simulink model "SistemaCompleto_PMSM"  (R2023b)
settings: Solver=VariableStepAuto  StartTime=0.0  StopTime=2  RelTol=1e-3
PostLoadFcn:
  | parametros_sistema_completo
  | run("parametros_sistema_completo.mlx")
values from neighbouring files (symbols this model uses):
  a_cu = 3.9e-3    (= 0.0039)    [parametros_sistema_completo.m]    (also in workspace_params.mat)
  A_i = [0,  1,                          0 ... (first row only)    [analisis_estabilidad_LA.m]
  b_eq = params.b_total    [calcular_matriz_AO.m]    (also in calculo_incertidumbre_y_control.m = b_m + b_l/(r^2); parametros_sistema_completo.m = 2.19444444444e-05; workspace_params.mat = 2.19444444444e-05)
  C_ts = C_ts * (1 + tol_pct)    [calculo_incertidumbre_y_control.m]    (also in parametros_sistema_completo.m = 0.818; workspace_params.mat = 0.818)
  g = 9.80665    [parametros_sistema_completo.m]    (also in workspace_params.mat)
  J_eq = params.J_total    [calcular_matriz_AO.m]    (also in calculo_incertidumbre_y_control.m = J_m + J_l/r^2; parametros_sistema_completo.m = 1.97847222222e-05; workspace_params.mat = 3.28055555556e-05)
  k_l = m*l_cm + m_l*l_l    [calculo_incertidumbre_y_control.m]    (also in parametros_sistema_completo.m = 0.25; workspace_params.mat = 0.625)
  L_d = L_d    * (1 - tol_pct)    [calculo_incertidumbre_y_control.m]    (also in parametros_sistema_completo.m = 0.0066; workspace_params.mat = 0.0066)
  L_ls = L_ls   * (1 - tol_pct)    [calculo_incertidumbre_y_control.m]    (also in parametros_sistema_completo.m = 0.0008; workspace_params.mat = 0.0008)
  L_q = L_q    * (1 - tol_pct)    [calculo_incertidumbre_y_control.m]    (also in parametros_sistema_completo.m = 0.0058; workspace_params.mat = 0.0058)
  lambda_r = lambda_r * (1 + tol_pct)    [calculo_incertidumbre_y_control.m]    (also in parametros_sistema_completo.m = 0.016; workspace_params.mat = 0.016)
  P_p = 3    [parametros_sistema_completo.m]    (also in workspace_params.mat)
  params = struct()    [evaluar_migracion_Ids.m]    (also in parametros_sistema_completo.m; workspace_params.mat = )
  r = params.r_red    [calcular_matriz_AO.m]    (also in parametros_sistema_completo.m = 120; workspace_params.mat = 120)
  R_s_sim = R_sREF * (1 + a_cu * (T_s_sim - T_sREF))    [configurar_temperatura_516.m]
  R_sREF = R_sREF * (1 - tol_pct)    [calculo_incertidumbre_y_control.m]    (also in parametros_sistema_completo.m = 1.02; workspace_params.mat = 1.02)
  R_ts_amb = R_ts_amb * (1 - tol_pct)    [calculo_incertidumbre_y_control.m]    (also in parametros_sistema_completo.m = 146.7; workspace_params.mat = 146.7)
  T_amb = 20    [parametros_sistema_completo.m]    (also in workspace_params.mat)
  T_s = x(6)    [modulador_torque_521.m]    (also in simulacion_dinamica_516.m)
  T_sREF = 20    [parametros_sistema_completo.m]    (also in workspace_params.mat)
undefined symbols (not defined in the file or in its folder): A_T, A_theta, A_v, b_a, B_i, B_T, B_theta, B_v, C_i, C_T, C_theta, C_v, consigna_posicion, D_i, D_T, D_theta, D_v, i_ds_inicial, Is_pico, Is_rms_max, Is_rms_nom, K_e_i_m_int, K_e_tita_m, K_e_tita_m_int, K_e_w_m, K_e_w_m_int, K_p0, K_pd, K_pq, K_sa, K_sia, pos_inicial, t_rampa_acel, t_rampa_vel, V_sl_max, x0_ias, x0_ibs, x0_ics, x0_T, x0_theta
libraries: simulink_extras x8, SignalEditorBlockLib x6, eeStairGenerator x4, simulink x1
(part 5 of 7)

== system SistemaCompleto_PMSM/Modelo Global NL Controlador modulador de torque3/Planta/Subsistema Electromagnetico ==
  v_qs : Inport
  v_ds : Inport  Port=2
  v_0s : Inport  Port=3
  ωm : Inport  Port=4
  R_s(T(t)) : Inport  Port=5
  Add : Sum  Inputs=-++
  Add1 : Sum  Inputs=--+
  Add2 : Sum  Inputs=|-+
  Add3 : Sum  Inputs=|++
  Gain : Gain  Gain=1/L_q
  Gain1 : Gain  Gain=1/L_d
  Gain2 : Gain  Gain=1/L_ls
  Gain3 : Gain  Gain=P_p
  Gain4 : Gain  Gain=L_d
  Gain5 : Gain  Gain=L_q
  Gain6 : Gain  Gain=3/2*P_p
  Gain7 : Gain  Gain=L_d-L_q
  Integrator : Integrator
  Integrator1 : Integrator  InitialCondition=i_ds_inicial
  Integrator2 : Integrator
  Product{,1..6} (7 alike) : Product
  Sum3 : Sum  Inputs=|++
  λ : Constant  Value=lambda_r
  i_qs : Outport
  i_ds : Outport  Port=2
  i_0s : Outport  Port=3
  T_m : Outport  Port=4
  wires:
  v_0s/1 -> Add2/2
  Gain5/1 -> Add/3
  Gain3/1 -> Product4/2, Product3/1  "ωr"
  Integrator/1 -> Product4/1, Product/2, i_qs/1, Product5/1, Product6/1
  v_qs/1 -> Add1/3
  R_s(T(t))/1 -> Product2/2, Product1/1, Product/1
  Gain4/1 -> Sum3/1
  Product1/1 -> Add/1
  Integrator2/1 -> i_0s/1, Product2/1
  Sum3/1 -> Product3/2
  Integrator1/1 -> Gain4/1, Product1/2, i_ds/1, Product6/2
  Product/1 -> Add1/2
  Product4/1 -> Gain5/1
  ωm/1 -> Gain3/1
  Add3/1 -> Gain6/1
  Gain/1 -> Integrator/1
  Gain6/1 -> T_m/1
  Product2/1 -> Add2/1
  λ/1 -> Sum3/2, Product5/2
  Gain1/1 -> Integrator1/1
  Add/1 -> Gain1/1
  Add1/1 -> Gain/1
  Product6/1 -> Gain7/1
  Product3/1 -> Add1/1
  Gain2/1 -> Integrator2/1
  Gain7/1 -> Add3/2
  v_ds/1 -> Add/2
  Add2/1 -> Gain2/1
  Product5/1 -> Add3/1

== system SistemaCompleto_PMSM/Modelo Global NL Controlador modulador de torque3/Planta/Subsistema Mecanico ==
  Tld(t)[N.m] : Inport
  Tm(t)[N.m] : Inport  Port=2
  1/J_eq[kg.m2] : Gain  Gain=1/J_eq
  Gain : Gain  Gain=1/r
  Gain1 : Gain  Gain=1/r
  Integrator : Integrator  InitialCondition=pos_inicial*r
  Integrator1 : Integrator
  Sin : Trigonometry
  Sum : Sum  Inputs=-+-
  Sum1 : Sum
  "[N.m/rad]" : Gain  Gain=g*k_l
  b_eq[N.m/rad/s] : Gain  Gain=b_eq
  θm(t) : Outport
  ωm(t) : Outport  Port=2
  wires:
  Gain1/1 -> Sin/1
  Sin/1 -> "[N.m/rad]"/1  "θm[rad]"
  Integrator1/1 -> Integrator/1, ωm(t)/1, b_eq[N.m/rad/s]/1  "ωm[rad/s]"
  Tld(t)[N.m]/1 -> Sum1/1
  b_eq[N.m/rad/s]/1 -> Sum/3
  1/J_eq[kg.m2]/1 -> Integrator1/1  "dω/dt [rad/s^2]"
  Gain/1 -> Sum/1
  "[N.m/rad]"/1 -> Sum1/2
  Integrator/1 -> θm(t)/1, Gain1/1  "θm[rad]"
  Sum/1 -> 1/J_eq[kg.m2]/1
  Tm(t)[N.m]/1 -> Sum/2
  Sum1/1 -> Gain/1

== system SistemaCompleto_PMSM/Modelo Global NL Controlador modulador de torque3/Planta/Subsistema Térmico ==
  i_qs2 : Inport
  i_ds2 : Inport  Port=2
  i_0s2 : Inport  Port=3
  Add : Sum  Inputs=+-
  Add1 : Sum
  Add2 : Sum  Inputs=+++
  Add3 : Sum  Inputs=+-
  Add4 : Sum  Inputs=-+
  Constant : Constant  Value=T_sREF
  Constant1 : Constant
  Constant2 : Constant  Value=T_amb
  Gain : Gain  Gain=R_sREF
  Gain1 : Gain  Gain=a_cu
  Gain2 : Gain  Gain=3/2
  Gain3 : Gain  Gain=2
  Gain4 : Gain  Gain=1/C_ts
  Gain5 : Gain  Gain=1/R_ts_amb
  Integrator : Integrator  InitialCondition=20
  Product : Product
  Square : Math  Operator=square  OutDataTypeStr=double
  Square1 : Math  Operator=square
  Square2 : Math  Operator=square
  R_s : Outport
  T_s : Outport  Port=2
  wires:
  Constant1/1 -> Add1/2
  Constant/1 -> Add/2
  i_qs2/1 -> Square/1
  Gain/1 -> R_s/1, Product/1
  Square/1 -> Add2/1
  Add2/1 -> Gain2/1
  Constant2/1 -> Add4/1
  i_ds2/1 -> Square1/1
  Gain5/1 -> Add3/2
  Integrator/1 -> Add4/2, T_s/1, Add/1  "T_s"
  Add1/1 -> Gain/1
  i_0s2/1 -> Square2/1
  Square1/1 -> Add2/2
  Product/1 -> Add3/1  "Ps_Perd"
  Gain2/1 -> Product/2
  Add/1 -> Gain1/1
  Square2/1 -> Gain3/1
  Gain1/1 -> Add1/1
  Add3/1 -> Gain4/1
  Add4/1 -> Gain5/1
  Gain3/1 -> Add2/3
  Gain4/1 -> Integrator/1

== system SistemaCompleto_PMSM/Modelo Global NL Controlador modulador de torque3/Planta/TI de Park ==
  f_q : Inport
  f_d : Inport  Port=2
  f_0 : Inport  Port=3
  θ_r : Inport  Port=4
  Add : Sum  Inputs=+++
  Add1 : Sum  Inputs=+-
  Add2 : Sum
  Add3 : Sum  Inputs=+++
  Add4 : Sum  Inputs=+++
  Constant : Constant  Value=2/3*pi
  Constant1 : Constant  Value=2/3*pi
  Cos : Trigonometry  Operator=cos
  Cos1 : Trigonometry
  Cos2 : Trigonometry  Operator=cos
  Cos3 : Trigonometry  Operator=cos
  Cos4 : Trigonometry
  Cos5 : Trigonometry
  Product{,1..5} (6 alike) : Product
  f_a : Outport
  f_b : Outport  Port=2
  f_c : Outport  Port=3
  wires:
  Product4/1 -> Add3/2
  Cos1/1 -> Product1/1
  Cos/1 -> Product/1
  Product1/1 -> Add/2
  Add3/1 -> f_b/1
  Cos3/1 -> Product3/1
  Product3/1 -> Add3/1
  f_d/1 -> Product1/2, Product5/2, Product4/2
  Constant1/1 -> Add2/2
  Constant/1 -> Add1/2
  f_0/1 -> Add3/3, Add4/3, Add/3
  Add1/1 -> Cos3/1, Cos4/1
  Product/1 -> Add/1
  f_q/1 -> Product/2, Product2/2, Product3/2
  Cos4/1 -> Product4/1
  θ_r/1 -> Add2/1, Add1/1, Cos/1, Cos1/1
  Add/1 -> f_a/1
  Add4/1 -> f_c/1
  Cos2/1 -> Product2/1
  Cos5/1 -> Product5/1
  Add2/1 -> Cos5/1, Cos2/1
  Product2/1 -> Add4/1
  Product5/1 -> Add4/2

== system SistemaCompleto_PMSM/Modelo Global NL Controlador modulador de torque3/Planta/Transformacion de Park ==
  f_a : Inport
  f_b : Inport  Port=2
  f_c : Inport  Port=3
  θ_r : Inport  Port=4
  Add : Sum  Inputs=+++
  Add1 : Sum  Inputs=+-
  Add2 : Sum
  Add3 : Sum  Inputs=+++
  Add4 : Sum  Inputs=+++
  Constant : Constant  Value=2/3*pi
  Constant1 : Constant  Value=2/3*pi
  Cos : Trigonometry  Operator=cos
  Cos1 : Trigonometry  Operator=cos
  Cos2 : Trigonometry  Operator=cos
  Cos3 : Trigonometry
  Cos4 : Trigonometry
  Cos5 : Trigonometry
  Gain1 : Gain  Gain=2/3
  Gain2 : Gain  Gain=2/3
  Gain3 : Gain  Gain=1/3
  Product{,1..5} (6 alike) : Product
  f_q : Outport
  f_d : Outport  Port=2
  f_0 : Outport  Port=3
  wires:
  Cos5/1 -> Product5/1
  Gain2/1 -> f_q/1
  Product5/1 -> Add3/3
  Add/1 -> Gain2/1
  θ_r/1 -> Cos3/1, Cos/1, Add1/1, Add2/1
  Cos4/1 -> Product4/1
  Cos2/1 -> Product2/1
  f_a/1 -> Add4/3, Product3/2, Product/2
  Product/1 -> Add/1
  Add1/1 -> Cos1/1, Cos4/1
  f_c/1 -> Product2/2, Product5/2, Add4/1
  Constant/1 -> Add1/2
  Constant1/1 -> Add2/2
  f_b/1 -> Product1/2, Product4/2, Add4/2
  Add2/1 -> Cos2/1, Cos5/1
  Add4/1 -> Gain3/1
  Product3/1 -> Add3/1
  Product2/1 -> Add/3
  Gain3/1 -> f_0/1
  Cos3/1 -> Product3/1
  Add3/1 -> Gain1/1
  Gain1/1 -> f_d/1
  Product1/1 -> Add/2
  Cos/1 -> Product/1
  Cos1/1 -> Product1/1
  Product4/1 -> Add3/2

== system SistemaCompleto_PMSM/Modelo Global NL Controlador modulador de torque4/Planta/Subsistema Electromagnetico ==
  v_qs : Inport
  v_ds : Inport  Port=2
  v_0s : Inport  Port=3
  ωm : Inport  Port=4
  R_s(T(t)) : Inport  Port=5
  Add : Sum  Inputs=-++
  Add1 : Sum  Inputs=--+
  Add2 : Sum  Inputs=|-+
  Add3 : Sum  Inputs=|++
  Gain : Gain  Gain=1/L_q
  Gain1 : Gain  Gain=1/L_d
  Gain2 : Gain  Gain=1/L_ls
  Gain3 : Gain  Gain=P_p
  Gain4 : Gain  Gain=L_d
  Gain5 : Gain  Gain=L_q
  Gain6 : Gain  Gain=3/2*P_p
  Gain7 : Gain  Gain=L_d-L_q
  Integrator : Integrator
  Integrator1 : Integrator  InitialCondition=i_ds_inicial
  Integrator2 : Integrator
  Product{,1..6} (7 alike) : Product
  Sum3 : Sum  Inputs=|++
  λ : Constant  Value=lambda_r
  i_qs : Outport
  i_ds : Outport  Port=2
  i_0s : Outport  Port=3
  T_m : Outport  Port=4
  wires:
  v_0s/1 -> Add2/2
  Gain5/1 -> Add/3
  Gain3/1 -> Product4/2, Product3/1  "ωr"
  Integrator/1 -> Product4/1, Product/2, i_qs/1, Product5/1, Product6/1
  v_qs/1 -> Add1/3
  R_s(T(t))/1 -> Product2/2, Product1/1, Product/1
  Gain4/1 -> Sum3/1
  Product1/1 -> Add/1
  Integrator2/1 -> i_0s/1, Product2/1
  Sum3/1 -> Product3/2
  Integrator1/1 -> Gain4/1, Product1/2, i_ds/1, Product6/2
  Product/1 -> Add1/2
  Product4/1 -> Gain5/1
  ωm/1 -> Gain3/1
  Add3/1 -> Gain6/1
  Gain/1 -> Integrator/1
  Gain6/1 -> T_m/1
  Product2/1 -> Add2/1
  λ/1 -> Sum3/2, Product5/2
  Gain1/1 -> Integrator1/1
  Add/1 -> Gain1/1
  Add1/1 -> Gain/1
  Product6/1 -> Gain7/1
  Product3/1 -> Add1/1
  Gain2/1 -> Integrator2/1
  Gain7/1 -> Add3/2
  v_ds/1 -> Add/2
  Add2/1 -> Gain2/1
  Product5/1 -> Add3/1

== system SistemaCompleto_PMSM/Modelo Global NL Controlador modulador de torque4/Planta/Subsistema Mecanico ==
  Tld(t)[N.m] : Inport
  Tm(t)[N.m] : Inport  Port=2
  1/J_eq[kg.m2] : Gain  Gain=1/J_eq
  Gain : Gain  Gain=1/r
  Gain1 : Gain  Gain=1/r
  Integrator : Integrator  InitialCondition=pos_inicial*r
  Integrator1 : Integrator
  Sin : Trigonometry
  Sum : Sum  Inputs=-+-
  Sum1 : Sum
  "[N.m/rad]" : Gain  Gain=g*k_l
  b_eq[N.m/rad/s] : Gain  Gain=b_eq
  θm(t) : Outport
  ωm(t) : Outport  Port=2
  wires:
  Gain1/1 -> Sin/1
  Sin/1 -> "[N.m/rad]"/1  "θm[rad]"
  Integrator1/1 -> Integrator/1, ωm(t)/1, b_eq[N.m/rad/s]/1  "ωm[rad/s]"
  Tld(t)[N.m]/1 -> Sum1/1
  b_eq[N.m/rad/s]/1 -> Sum/3
  1/J_eq[kg.m2]/1 -> Integrator1/1  "dω/dt [rad/s^2]"
  Gain/1 -> Sum/1
  "[N.m/rad]"/1 -> Sum1/2
  Integrator/1 -> θm(t)/1, Gain1/1  "θm[rad]"
  Sum/1 -> 1/J_eq[kg.m2]/1
  Tm(t)[N.m]/1 -> Sum/2
  Sum1/1 -> Gain/1

== system SistemaCompleto_PMSM/Modelo Global NL Controlador modulador de torque4/Planta/Subsistema Térmico ==
  i_qs2 : Inport
  i_ds2 : Inport  Port=2
  i_0s2 : Inport  Port=3
  Add : Sum  Inputs=+-
  Add1 : Sum
  Add2 : Sum  Inputs=+++
  Add3 : Sum  Inputs=+-
  Add4 : Sum  Inputs=-+
  Constant : Constant  Value=T_sREF
  Constant1 : Constant
  Constant2 : Constant  Value=T_amb
  Gain : Gain  Gain=R_sREF
  Gain1 : Gain  Gain=a_cu
  Gain2 : Gain  Gain=3/2
  Gain3 : Gain  Gain=2
  Gain4 : Gain  Gain=1/C_ts
  Gain5 : Gain  Gain=1/R_ts_amb
  Integrator : Integrator  InitialCondition=20
  Product : Product
  Square : Math  Operator=square  OutDataTypeStr=double
  Square1 : Math  Operator=square
  Square2 : Math  Operator=square
  R_s : Outport
  T_s : Outport  Port=2
  wires:
  Constant1/1 -> Add1/2
  Constant/1 -> Add/2
  i_qs2/1 -> Square/1
  Gain/1 -> R_s/1, Product/1
  Square/1 -> Add2/1
  Add2/1 -> Gain2/1
  Constant2/1 -> Add4/1
  i_ds2/1 -> Square1/1
  Gain5/1 -> Add3/2
  Integrator/1 -> Add4/2, T_s/1, Add/1  "T_s"
  Add1/1 -> Gain/1
  i_0s2/1 -> Square2/1
  Square1/1 -> Add2/2
  Product/1 -> Add3/1  "Ps_Perd"
  Gain2/1 -> Product/2
  Add/1 -> Gain1/1
  Square2/1 -> Gain3/1
  Gain1/1 -> Add1/1
  Add3/1 -> Gain4/1
  Add4/1 -> Gain5/1
  Gain3/1 -> Add2/3
  Gain4/1 -> Integrator/1

== system SistemaCompleto_PMSM/Modelo Global NL Controlador modulador de torque4/Planta/TI de Park ==
  f_q : Inport
  f_d : Inport  Port=2
  f_0 : Inport  Port=3
  θ_r : Inport  Port=4
  Add : Sum  Inputs=+++
  Add1 : Sum  Inputs=+-
  Add2 : Sum
  Add3 : Sum  Inputs=+++
  Add4 : Sum  Inputs=+++
  Constant : Constant  Value=2/3*pi
  Constant1 : Constant  Value=2/3*pi
  Cos : Trigonometry  Operator=cos
  Cos1 : Trigonometry
  Cos2 : Trigonometry  Operator=cos
  Cos3 : Trigonometry  Operator=cos
  Cos4 : Trigonometry
  Cos5 : Trigonometry
  Product{,1..5} (6 alike) : Product
  f_a : Outport
  f_b : Outport  Port=2
  f_c : Outport  Port=3
  wires:
  Product4/1 -> Add3/2
  Cos1/1 -> Product1/1
  Cos/1 -> Product/1
  Product1/1 -> Add/2
  Add3/1 -> f_b/1
  Cos3/1 -> Product3/1
  Product3/1 -> Add3/1
  f_d/1 -> Product1/2, Product5/2, Product4/2
  Constant1/1 -> Add2/2
  Constant/1 -> Add1/2
  f_0/1 -> Add3/3, Add4/3, Add/3
  Add1/1 -> Cos3/1, Cos4/1
  Product/1 -> Add/1
  f_q/1 -> Product/2, Product2/2, Product3/2
  Cos4/1 -> Product4/1
  θ_r/1 -> Add2/1, Add1/1, Cos/1, Cos1/1
  Add/1 -> f_a/1
  Add4/1 -> f_c/1
  Cos2/1 -> Product2/1
  Cos5/1 -> Product5/1
  Add2/1 -> Cos5/1, Cos2/1
  Product2/1 -> Add4/1
  Product5/1 -> Add4/2

== system SistemaCompleto_PMSM/Modelo Global NL Controlador modulador de torque4/Planta/Transformacion de Park ==
  f_a : Inport
  f_b : Inport  Port=2
  f_c : Inport  Port=3
  θ_r : Inport  Port=4
  Add : Sum  Inputs=+++
  Add1 : Sum  Inputs=+-
  Add2 : Sum
  Add3 : Sum  Inputs=+++
  Add4 : Sum  Inputs=+++
  Constant : Constant  Value=2/3*pi
  Constant1 : Constant  Value=2/3*pi
  Cos : Trigonometry  Operator=cos
  Cos1 : Trigonometry  Operator=cos
  Cos2 : Trigonometry  Operator=cos
  Cos3 : Trigonometry
  Cos4 : Trigonometry
  Cos5 : Trigonometry
  Gain1 : Gain  Gain=2/3
  Gain2 : Gain  Gain=2/3
  Gain3 : Gain  Gain=1/3
  Product{,1..5} (6 alike) : Product
  f_q : Outport
  f_d : Outport  Port=2
  f_0 : Outport  Port=3
  wires:
  Cos5/1 -> Product5/1
  Gain2/1 -> f_q/1
  Product5/1 -> Add3/3
  Add/1 -> Gain2/1
  θ_r/1 -> Cos3/1, Cos/1, Add1/1, Add2/1
  Cos4/1 -> Product4/1
  Cos2/1 -> Product2/1
  f_a/1 -> Add4/3, Product3/2, Product/2
  Product/1 -> Add/1
  Add1/1 -> Cos1/1, Cos4/1
  f_c/1 -> Product2/2, Product5/2, Add4/1
  Constant/1 -> Add1/2
  Constant1/1 -> Add2/2
  f_b/1 -> Product1/2, Product4/2, Add4/2
  Add2/1 -> Cos2/1, Cos5/1
  Add4/1 -> Gain3/1
  Product3/1 -> Add3/1
  Product2/1 -> Add/3
  Gain3/1 -> f_0/1
  Cos3/1 -> Product3/1
  Add3/1 -> Gain1/1
  Gain1/1 -> f_d/1
  Product1/1 -> Add/2
  Cos/1 -> Product/1
  Cos1/1 -> Product1/1
  Product4/1 -> Add3/2

== system SistemaCompleto_PMSM/Modelo Global NL perfil trapezoidal aceleracion/Planta/Subsistema Electromagnetico ==
  v_qs : Inport
  v_ds : Inport  Port=2
  v_0s : Inport  Port=3
  ωm : Inport  Port=4
  R_s(T(t)) : Inport  Port=5
  Add : Sum  Inputs=-++
  Add1 : Sum  Inputs=--+
  Add2 : Sum  Inputs=|-+
  Add3 : Sum  Inputs=|++
  Gain : Gain  Gain=1/L_q
  Gain1 : Gain  Gain=1/L_d
  Gain2 : Gain  Gain=1/L_ls
  Gain3 : Gain  Gain=P_p
  Gain4 : Gain  Gain=L_d
  Gain5 : Gain  Gain=L_q
  Gain6 : Gain  Gain=3/2*P_p
  Gain7 : Gain  Gain=L_d-L_q
  Integrator : Integrator
  Integrator1 : Integrator  InitialCondition=i_ds_inicial
  Integrator2 : Integrator
  Product{,1..6} (7 alike) : Product
  Sum3 : Sum  Inputs=|++
  λ : Constant  Value=lambda_r
  i_qs : Outport
  i_ds : Outport  Port=2
  i_0s : Outport  Port=3
  T_m : Outport  Port=4
  wires:
  v_0s/1 -> Add2/2
  Gain5/1 -> Add/3
  Gain3/1 -> Product4/2, Product3/1  "ωr"
  Integrator/1 -> Product4/1, Product/2, i_qs/1, Product5/1, Product6/1
  v_qs/1 -> Add1/3
  R_s(T(t))/1 -> Product2/2, Product1/1, Product/1
  Gain4/1 -> Sum3/1
  Product1/1 -> Add/1
  Integrator2/1 -> i_0s/1, Product2/1
  Sum3/1 -> Product3/2
  Integrator1/1 -> Gain4/1, Product1/2, i_ds/1, Product6/2
  Product/1 -> Add1/2
  Product4/1 -> Gain5/1
  ωm/1 -> Gain3/1
  Add3/1 -> Gain6/1
  Gain/1 -> Integrator/1
  Gain6/1 -> T_m/1
  Product2/1 -> Add2/1
  λ/1 -> Sum3/2, Product5/2
  Gain1/1 -> Integrator1/1
  Add/1 -> Gain1/1
  Add1/1 -> Gain/1
  Product6/1 -> Gain7/1
  Product3/1 -> Add1/1
  Gain2/1 -> Integrator2/1
  Gain7/1 -> Add3/2
  v_ds/1 -> Add/2
  Add2/1 -> Gain2/1
  Product5/1 -> Add3/1

== system SistemaCompleto_PMSM/Modelo Global NL perfil trapezoidal aceleracion/Planta/Subsistema Mecanico ==
  Tld(t)[N.m] : Inport
  Tm(t)[N.m] : Inport  Port=2
  1/J_eq[kg.m2] : Gain  Gain=1/J_eq
  Gain : Gain  Gain=1/r
  Gain1 : Gain  Gain=1/r
  Integrator : Integrator  InitialCondition=pos_inicial*r
  Integrator1 : Integrator
  Sin : Trigonometry
  Sum : Sum  Inputs=-+-
  Sum1 : Sum
  "[N.m/rad]" : Gain  Gain=g*k_l
  b_eq[N.m/rad/s] : Gain  Gain=b_eq
  θm(t) : Outport
  ωm(t) : Outport  Port=2
  wires:
  Gain1/1 -> Sin/1
  Sin/1 -> "[N.m/rad]"/1  "θm[rad]"
  Integrator1/1 -> Integrator/1, ωm(t)/1, b_eq[N.m/rad/s]/1  "ωm[rad/s]"
  Tld(t)[N.m]/1 -> Sum1/1
  b_eq[N.m/rad/s]/1 -> Sum/3
  1/J_eq[kg.m2]/1 -> Integrator1/1  "dω/dt [rad/s^2]"
  Gain/1 -> Sum/1
  "[N.m/rad]"/1 -> Sum1/2
  Integrator/1 -> θm(t)/1, Gain1/1  "θm[rad]"
  Sum/1 -> 1/J_eq[kg.m2]/1
  Tm(t)[N.m]/1 -> Sum/2
  Sum1/1 -> Gain/1

== system SistemaCompleto_PMSM/Modelo Global NL perfil trapezoidal aceleracion/Planta/Subsistema Térmico ==
  i_qs2 : Inport
  i_ds2 : Inport  Port=2
  i_0s2 : Inport  Port=3
  Add : Sum  Inputs=+-
  Add1 : Sum
  Add2 : Sum  Inputs=+++
  Add3 : Sum  Inputs=+-
  Add4 : Sum  Inputs=-+
  Constant : Constant  Value=T_sREF
  Constant1 : Constant
  Constant2 : Constant  Value=T_amb
  Gain : Gain  Gain=R_sREF
  Gain1 : Gain  Gain=a_cu
  Gain2 : Gain  Gain=3/2
  Gain3 : Gain  Gain=2
  Gain4 : Gain  Gain=1/C_ts
  Gain5 : Gain  Gain=1/R_ts_amb
  Integrator : Integrator  InitialCondition=T_amb
  Product : Product
  Square : Math  Operator=square  OutDataTypeStr=double
  Square1 : Math  Operator=square
  Square2 : Math  Operator=square
  R_s : Outport
  T_s : Outport  Port=2
  wires:
  Constant1/1 -> Add1/2
  Constant/1 -> Add/2
  i_qs2/1 -> Square/1
  Gain/1 -> R_s/1, Product/1
  Square/1 -> Add2/1
  Add2/1 -> Gain2/1
  Constant2/1 -> Add4/1
  i_ds2/1 -> Square1/1
  Gain5/1 -> Add3/2
  Integrator/1 -> Add4/2, T_s/1, Add/1  "T_s"
  Add1/1 -> Gain/1
  i_0s2/1 -> Square2/1
  Square1/1 -> Add2/2
  Product/1 -> Add3/1  "Ps_Perd"
  Gain2/1 -> Product/2
  Add/1 -> Gain1/1
  Square2/1 -> Gain3/1
  Gain1/1 -> Add1/1
  Add3/1 -> Gain4/1
  Add4/1 -> Gain5/1
  Gain3/1 -> Add2/3
  Gain4/1 -> Integrator/1

== system SistemaCompleto_PMSM/Modelo Global NL perfil trapezoidal aceleracion/Planta/TI de Park ==
  f_q : Inport
  f_d : Inport  Port=2
  f_0 : Inport  Port=3
  θ_r : Inport  Port=4
  Add : Sum  Inputs=+++
  Add1 : Sum  Inputs=+-
  Add2 : Sum
  Add3 : Sum  Inputs=+++
  Add4 : Sum  Inputs=+++
  Constant : Constant  Value=2/3*pi
  Constant1 : Constant  Value=2/3*pi
  Cos : Trigonometry  Operator=cos
  Cos1 : Trigonometry
  Cos2 : Trigonometry  Operator=cos
  Cos3 : Trigonometry  Operator=cos
  Cos4 : Trigonometry
  Cos5 : Trigonometry
  Product{,1..5} (6 alike) : Product
  f_a : Outport
  f_b : Outport  Port=2
  f_c : Outport  Port=3
  wires:
  Product4/1 -> Add3/2
  Cos1/1 -> Product1/1
  Cos/1 -> Product/1
  Product1/1 -> Add/2
  Add3/1 -> f_b/1
  Cos3/1 -> Product3/1
  Product3/1 -> Add3/1
  f_d/1 -> Product1/2, Product5/2, Product4/2
  Constant1/1 -> Add2/2
  Constant/1 -> Add1/2
  f_0/1 -> Add3/3, Add4/3, Add/3
  Add1/1 -> Cos3/1, Cos4/1
  Product/1 -> Add/1
  f_q/1 -> Product/2, Product2/2, Product3/2
  Cos4/1 -> Product4/1
  θ_r/1 -> Add2/1, Add1/1, Cos/1, Cos1/1
  Add/1 -> f_a/1
  Add4/1 -> f_c/1
  Cos2/1 -> Product2/1
  Cos5/1 -> Product5/1
  Add2/1 -> Cos5/1, Cos2/1
  Product2/1 -> Add4/1
  Product5/1 -> Add4/2

== system SistemaCompleto_PMSM/Modelo Global NL perfil trapezoidal aceleracion/Planta/Transformacion de Park ==
  f_a : Inport
  f_b : Inport  Port=2
  f_c : Inport  Port=3
  θ_r : Inport  Port=4
  Add : Sum  Inputs=+++
  Add1 : Sum  Inputs=+-
  Add2 : Sum
  Add3 : Sum  Inputs=+++
  Add4 : Sum  Inputs=+++
  Constant : Constant  Value=2/3*pi
  Constant1 : Constant  Value=2/3*pi
  Cos : Trigonometry  Operator=cos
  Cos1 : Trigonometry  Operator=cos
  Cos2 : Trigonometry  Operator=cos
  Cos3 : Trigonometry
  Cos4 : Trigonometry
  Cos5 : Trigonometry
  Gain1 : Gain  Gain=2/3
  Gain2 : Gain  Gain=2/3
  Gain3 : Gain  Gain=1/3
  Product{,1..5} (6 alike) : Product
  f_q : Outport
  f_d : Outport  Port=2
  f_0 : Outport  Port=3
  wires:
  Cos5/1 -> Product5/1
  Gain2/1 -> f_q/1
  Product5/1 -> Add3/3
  Add/1 -> Gain2/1
  θ_r/1 -> Cos3/1, Cos/1, Add1/1, Add2/1
  Cos4/1 -> Product4/1
  Cos2/1 -> Product2/1
  f_a/1 -> Add4/3, Product3/2, Product/2
  Product/1 -> Add/1
  Add1/1 -> Cos1/1, Cos4/1
  f_c/1 -> Product2/2, Product5/2, Add4/1
  Constant/1 -> Add1/2
  Constant1/1 -> Add2/2
  f_b/1 -> Product1/2, Product4/2, Add4/2
  Add2/1 -> Cos2/1, Cos5/1
  Add4/1 -> Gain3/1
  Product3/1 -> Add3/1
  Product2/1 -> Add/3
  Gain3/1 -> f_0/1
  Cos3/1 -> Product3/1
  Add3/1 -> Gain1/1
  Gain1/1 -> f_d/1
  Product1/1 -> Add/2
  Cos/1 -> Product/1
  Cos1/1 -> Product1/1
  Product4/1 -> Add3/2

== system SistemaCompleto_PMSM/Modelo Global NL perfil trapezoidal aceleracion y codificado/Controlador/Controlador PID de Posicion ==
  ωm[rad/s] : Inport
  ωm*[rad/s] : Inport  Port=2
  Constant : Constant  Value=params  OutDataTypeStr=Bus: ParamsBus
  MATLAB Function1 : MATLAB Function  TreatAsAtomicUnit=on
  Sum1 : Sum  Inputs=-+|
  Zero-Order Hold1 : ZeroOrderHold  SampleTime=T_s
  Zero-Order Hold2 : ZeroOrderHold  SampleTime=T_s
  Tm*' : Outport
  wires:
  Zero-Order Hold1/1 -> MATLAB Function1/1(e_wm)
  ωm[rad/s]/1 -> Sum1/1
  ωm*[rad/s]/1 -> Sum1/2
  MATLAB Function1/1(Tm) -> Zero-Order Hold2/1
  Zero-Order Hold2/1 -> Tm*'/1
  Sum1/1 -> Zero-Order Hold1/1  "eωm"
  Constant/1 -> MATLAB Function1/2(params)

== system SistemaCompleto_PMSM/Modelo Global NL perfil trapezoidal aceleracion y codificado/Controlador/Desacople de Realimentaciones Fisicas Naturales ==
  R_s : Inport
  ωm : Inport  Port=2
  i_qs : Inport  Port=3
  v_qs* : Inport  Port=4
  v_ds* : Inport  Port=5
  v_0s* : Inport  Port=6
  i_0s : Inport  Port=7
  i_ds : Inport  Port=8
  Constant : Constant  Value=params  OutDataTypeStr=Bus: ParamsBus
  MATLAB Function : MATLAB Function  TreatAsAtomicUnit=on
  v_qs [V] : Outport
  v_ds [V] : Outport  Port=2
  v_0s [V] : Outport  Port=3
  wires:
  v_qs*/1 -> MATLAB Function/1(v_qs_ref)
  R_s/1 -> MATLAB Function/2(Rs)
  ωm/1 -> MATLAB Function/3(wm)
  v_ds*/1 -> MATLAB Function/4(v_ds_ref)
  v_0s*/1 -> MATLAB Function/5(v_0s_ref)
  i_0s/1 -> MATLAB Function/6(i_0s)
  i_qs/1 -> MATLAB Function/7(i_qs)
  i_ds/1 -> MATLAB Function/8(i_ds)
  Constant/1 -> MATLAB Function/9(params)
  MATLAB Function/1(v_qs) -> v_qs [V]/1
  MATLAB Function/2(v_ds) -> v_ds [V]/1
  MATLAB Function/3(v_0s) -> v_0s [V]/1

== system SistemaCompleto_PMSM/Modelo Global NL perfil trapezoidal aceleracion y codificado/Controlador/Modulador de Corriente ==
  i_qs : Inport
  i_qs* : Inport  Port=2
  i_ds* : Inport  Port=3
  i_ds : Inport  Port=4
  i_0s* : Inport  Port=5
  i_0s : Inport  Port=6
  Constant : Constant  Value=params  OutDataTypeStr=Bus: ParamsBus
  MATLAB Function : MATLAB Function  TreatAsAtomicUnit=on
  v_qs* : Outport
  v_ds* : Outport  Port=2
  v_0s* : Outport  Port=3
  wires:
  i_qs*/1 -> MATLAB Function/1(i_qs_ref)
  i_qs/1 -> MATLAB Function/2(i_qs)
  i_ds*/1 -> MATLAB Function/3(i_ds_ref)
  i_ds/1 -> MATLAB Function/4(i_ds)
  i_0s*/1 -> MATLAB Function/5(i_0s_ref)
  i_0s/1 -> MATLAB Function/6(i_0s)
  Constant/1 -> MATLAB Function/7(params)
  MATLAB Function/1(v_qs_ref) -> v_qs*/1
  MATLAB Function/2(v_ds_ref) -> v_ds*/1
  MATLAB Function/3(v_0s_ref) -> v_0s*/1

== system SistemaCompleto_PMSM/Modelo Global NL perfil trapezoidal aceleracion y codificado/Controlador/Modulador de Torque ==
  ωm[rad/s] : Inport
  θm [rad] : Inport  Port=2
  T_m*'[N.m] : Inport  Port=3
  i_ds [A] : Inport  Port=4
  g[m/s2] : Inport  Port=5
  Constant1 : Constant  Value=params  OutDataTypeStr=Bus: ParamsBus
  MATLAB Function : MATLAB Function  TreatAsAtomicUnit=on
  i_qs* : Outport
  wires:
  T_m*'[N.m]/1 -> MATLAB Function/1(Tm_ref)
  ωm[rad/s]/1 -> MATLAB Function/2(wm)
  MATLAB Function/1(i_qs_ref) -> i_qs*/1
  θm [rad]/1 -> MATLAB Function/3(theta_m)
  i_ds [A]/1 -> MATLAB Function/4(i_ds)
  g[m/s2]/1 -> MATLAB Function/5(g)
  Constant1/1 -> MATLAB Function/6(params)

== system SistemaCompleto_PMSM/Modelo Global NL perfil trapezoidal aceleracion y codificado/Controlador/Observador de Estado de velocidad  ==
  θ : Inport
  Te*' : Inport  Port=2
  Constant : Constant  Value=params  OutDataTypeStr=Bus: ParamsBus  LockScale=on
  MATLAB Function : MATLAB Function  TreatAsAtomicUnit=on
  Unit Delay : UnitDelay  SampleTime=T_s  HasFrameUpgradeWarning=on
  Zero-Order Hold1 : ZeroOrderHold  SampleTime=T_s
  Zero-Order Hold2 : ZeroOrderHold  SampleTime=T_s
  ω~ : Outport
  wires:
  θ/1 -> Zero-Order Hold2/1
  Zero-Order Hold2/1 -> MATLAB Function/1(theta)
  Constant/1 -> MATLAB Function/3(params)
  MATLAB Function/1(wm_est) -> ω~/1
  Te*'/1 -> Unit Delay/1
  Zero-Order Hold1/1 -> MATLAB Function/2(Te_ref)
  Unit Delay/1 -> Zero-Order Hold1/1

== system SistemaCompleto_PMSM/Modelo Global NL perfil trapezoidal aceleracion y codificado/Controlador/T. Directa de Park ==
  f_a : Inport
  f_b : Inport  Port=2
  f_c : Inport  Port=3
  θ_r : Inport  Port=4
  Constant : Constant  Value=params  OutDataTypeStr=Bus: ParamsBus
  MATLAB Function : MATLAB Function  TreatAsAtomicUnit=on
  f_q : Outport
  f_d : Outport  Port=2
  f_0 : Outport  Port=3
  wires:
  MATLAB Function/2(f_d) -> f_d/1
  MATLAB Function/1(f_q) -> f_q/1
  f_a/1 -> MATLAB Function/1(f_a)
  MATLAB Function/3(f_0) -> f_0/1
  f_b/1 -> MATLAB Function/2(f_b)
  f_c/1 -> MATLAB Function/3(f_c)
  θ_r/1 -> MATLAB Function/4(theta_m)
  Constant/1 -> MATLAB Function/5(params)

== system SistemaCompleto_PMSM/Modelo Global NL perfil trapezoidal aceleracion y codificado/Controlador/T. Inversa de Park ==
  θ_r : Inport
  f_q : Inport  Port=2
  f_d : Inport  Port=3
  f_0 : Inport  Port=4
  Constant : Constant  Value=params  OutDataTypeStr=Bus: ParamsBus
  MATLAB Function : MATLAB Function  TreatAsAtomicUnit=on
  f_a : Outport
  f_b : Outport  Port=2
  f_c : Outport  Port=3
  wires:
  MATLAB Function/3(f_c) -> f_c/1
  f_q/1 -> MATLAB Function/1(f_q)
  f_d/1 -> MATLAB Function/2(f_d)
  f_0/1 -> MATLAB Function/3(f_0)
  MATLAB Function/2(f_b) -> f_b/1
  MATLAB Function/1(f_a) -> f_a/1
  θ_r/1 -> MATLAB Function/4(theta_m)
  Constant/1 -> MATLAB Function/5(params)

== system SistemaCompleto_PMSM/Modelo Global NL perfil trapezoidal aceleracion y codificado/Planta/Subsistema Electromagnetico ==
  v_qs : Inport
  v_ds : Inport  Port=2
  v_0s : Inport  Port=3
  ωm : Inport  Port=4
  R_s(T(t)) : Inport  Port=5
  Add : Sum  Inputs=-++
  Add1 : Sum  Inputs=--+
  Add2 : Sum  Inputs=|-+
  Add3 : Sum  Inputs=|++
  Gain : Gain  Gain=1/L_q
  Gain1 : Gain  Gain=1/L_d
  Gain2 : Gain  Gain=1/L_ls
  Gain3 : Gain  Gain=P_p
  Gain4 : Gain  Gain=L_d
  Gain5 : Gain  Gain=L_q
  Gain6 : Gain  Gain=3/2*P_p
  Gain7 : Gain  Gain=L_d-L_q
  Integrator : Integrator
  Integrator1 : Integrator  InitialCondition=i_ds_inicial
  Integrator2 : Integrator
  Product{,1..6} (7 alike) : Product
  Sum3 : Sum  Inputs=|++
  λ : Constant  Value=lambda_r
  i_qs : Outport
  i_ds : Outport  Port=2
  i_0s : Outport  Port=3
  T_m : Outport  Port=4
  wires:
  v_0s/1 -> Add2/2
  Gain5/1 -> Add/3
  Gain3/1 -> Product4/2, Product3/1  "ωr"
  Integrator/1 -> Product4/1, Product/2, i_qs/1, Product5/1, Product6/1
  v_qs/1 -> Add1/3
  R_s(T(t))/1 -> Product2/2, Product1/1, Product/1
  Gain4/1 -> Sum3/1
  Product1/1 -> Add/1
  Integrator2/1 -> i_0s/1, Product2/1
  Sum3/1 -> Product3/2
  Integrator1/1 -> Gain4/1, Product1/2, i_ds/1, Product6/2
  Product/1 -> Add1/2
  Product4/1 -> Gain5/1
  ωm/1 -> Gain3/1
  Add3/1 -> Gain6/1
  Gain/1 -> Integrator/1
  Gain6/1 -> T_m/1
  Product2/1 -> Add2/1
  λ/1 -> Sum3/2, Product5/2
  Gain1/1 -> Integrator1/1
  Add/1 -> Gain1/1
  Add1/1 -> Gain/1
  Product6/1 -> Gain7/1
  Product3/1 -> Add1/1
  Gain2/1 -> Integrator2/1
  Gain7/1 -> Add3/2
  v_ds/1 -> Add/2
  Add2/1 -> Gain2/1
  Product5/1 -> Add3/1

== system SistemaCompleto_PMSM/Modelo Global NL perfil trapezoidal aceleracion y codificado/Planta/Subsistema Mecanico ==
  Tld(t)[N.m] : Inport
  Tm(t)[N.m] : Inport  Port=2
  g [m/s2] : Inport  Port=3
  1/J_eq[kg.m2] : Gain  Gain=1/J_eq
  Gain : Gain  Gain=1/r
  Gain1 : Gain  Gain=1/r
  Integrator : Integrator  InitialCondition=pos_inicial*r
  Integrator1 : Integrator
  Product : Product
  Sin : Trigonometry
  Sum : Sum  Inputs=-+-
  Sum1 : Sum
  "[N.m/rad]" : Gain  Gain=k_l
  b_eq[N.m/rad/s] : Gain  Gain=b_eq
  θm(t) : Outport
  ωm(t) : Outport  Port=2
  wires:
  Gain1/1 -> Sin/1
  Sin/1 -> "[N.m/rad]"/1  "θm[rad]"
  Integrator1/1 -> Integrator/1, ωm(t)/1, b_eq[N.m/rad/s]/1  "ωm[rad/s]"
  Tld(t)[N.m]/1 -> Sum1/1
  b_eq[N.m/rad/s]/1 -> Sum/3
  1/J_eq[kg.m2]/1 -> Integrator1/1  "dω/dt [rad/s^2]"
  Gain/1 -> Sum/1
  Integrator/1 -> Gain1/1, θm(t)/1  "θm[rad]"
  Sum/1 -> 1/J_eq[kg.m2]/1
  Tm(t)[N.m]/1 -> Sum/2
  Sum1/1 -> Gain/1
  g [m/s2]/1 -> Product/1
  Product/1 -> Sum1/2
  "[N.m/rad]"/1 -> Product/2

== system SistemaCompleto_PMSM/Modelo Global NL perfil trapezoidal aceleracion y codificado/Planta/Subsistema Térmico ==
  i_qs2 : Inport
  i_ds2 : Inport  Port=2
  i_0s2 : Inport  Port=3
  Add : Sum  Inputs=+-
  Add1 : Sum
  Add2 : Sum  Inputs=+++
  Add3 : Sum  Inputs=+-
  Add4 : Sum  Inputs=-+
  Constant : Constant  Value=T_sREF
  Constant1 : Constant
  Constant2 : Constant  Value=T_amb
  Gain : Gain  Gain=R_sREF
  Gain1 : Gain  Gain=a_cu
  Gain2 : Gain  Gain=3/2
  Gain3 : Gain  Gain=2
  Gain4 : Gain  Gain=1/C_ts
  Gain5 : Gain  Gain=1/R_ts_amb
  Integrator : Integrator  InitialCondition=T_amb
  Product : Product
  Square : Math  Operator=square  OutDataTypeStr=double
  Square1 : Math  Operator=square
  Square2 : Math  Operator=square
  R_s : Outport
  T_s : Outport  Port=2
  wires:
  Constant1/1 -> Add1/2
  Constant/1 -> Add/2
  i_qs2/1 -> Square/1
  Gain/1 -> R_s/1, Product/1
  Square/1 -> Add2/1
  Add2/1 -> Gain2/1
  Constant2/1 -> Add4/1
  i_ds2/1 -> Square1/1
  Gain5/1 -> Add3/2
  Integrator/1 -> Add4/2, T_s/1, Add/1  "T_s"
  Add1/1 -> Gain/1
  i_0s2/1 -> Square2/1
  Square1/1 -> Add2/2
  Product/1 -> Add3/1  "Ps_Perd"
  Gain2/1 -> Product/2
  Add/1 -> Gain1/1
  Square2/1 -> Gain3/1
  Gain1/1 -> Add1/1
  Add3/1 -> Gain4/1
  Add4/1 -> Gain5/1
  Gain3/1 -> Add2/3
  Gain4/1 -> Integrator/1

== system SistemaCompleto_PMSM/Modelo Global NL perfil trapezoidal aceleracion y codificado/Planta/TI de Park ==
  f_q : Inport
  f_d : Inport  Port=2
  f_0 : Inport  Port=3
  θ_r : Inport  Port=4
  Add : Sum  Inputs=+++
  Add1 : Sum  Inputs=+-
  Add2 : Sum
  Add3 : Sum  Inputs=+++
  Add4 : Sum  Inputs=+++
  Constant : Constant  Value=2/3*pi
  Constant1 : Constant  Value=2/3*pi
  Cos : Trigonometry  Operator=cos
  Cos1 : Trigonometry
  Cos2 : Trigonometry  Operator=cos
  Cos3 : Trigonometry  Operator=cos
  Cos4 : Trigonometry
  Cos5 : Trigonometry
  Product{,1..5} (6 alike) : Product
  f_a : Outport
  f_b : Outport  Port=2
  f_c : Outport  Port=3
  wires:
  Product4/1 -> Add3/2
  Cos1/1 -> Product1/1
  Cos/1 -> Product/1
  Product1/1 -> Add/2
  Add3/1 -> f_b/1
  Cos3/1 -> Product3/1
  Product3/1 -> Add3/1
  f_d/1 -> Product1/2, Product5/2, Product4/2
  Constant1/1 -> Add2/2
  Constant/1 -> Add1/2
  f_0/1 -> Add3/3, Add4/3, Add/3
  Add1/1 -> Cos3/1, Cos4/1
  Product/1 -> Add/1
  f_q/1 -> Product/2, Product2/2, Product3/2
  Cos4/1 -> Product4/1
  θ_r/1 -> Add2/1, Add1/1, Cos/1, Cos1/1
  Add/1 -> f_a/1
  Add4/1 -> f_c/1
  Cos2/1 -> Product2/1
  Cos5/1 -> Product5/1
  Add2/1 -> Cos5/1, Cos2/1
  Product2/1 -> Add4/1
  Product5/1 -> Add4/2

== system SistemaCompleto_PMSM/Modelo Global NL perfil trapezoidal aceleracion y codificado/Planta/Transformacion de Park ==
  f_a : Inport
  f_b : Inport  Port=2
  f_c : Inport  Port=3
  θ_r : Inport  Port=4
  Add : Sum  Inputs=+++
  Add1 : Sum  Inputs=+-
  Add2 : Sum
  Add3 : Sum  Inputs=+++
  Add4 : Sum  Inputs=+++
  Constant : Constant  Value=2/3*pi
  Constant1 : Constant  Value=2/3*pi
  Cos : Trigonometry  Operator=cos
  Cos1 : Trigonometry  Operator=cos
  Cos2 : Trigonometry  Operator=cos
  Cos3 : Trigonometry
  Cos4 : Trigonometry
  Cos5 : Trigonometry
  Gain1 : Gain  Gain=2/3
  Gain2 : Gain  Gain=2/3
  Gain3 : Gain  Gain=1/3
  Product{,1..5} (6 alike) : Product
  f_q : Outport
  f_d : Outport  Port=2
  f_0 : Outport  Port=3
  wires:
  Cos5/1 -> Product5/1
  Gain2/1 -> f_q/1
  Product5/1 -> Add3/3
  Add/1 -> Gain2/1
  θ_r/1 -> Cos3/1, Cos/1, Add1/1, Add2/1
  Cos4/1 -> Product4/1
  Cos2/1 -> Product2/1
  f_a/1 -> Add4/3, Product3/2, Product/2
  Product/1 -> Add/1
  Add1/1 -> Cos1/1, Cos4/1
  f_c/1 -> Product2/2, Product5/2, Add4/1
  Constant/1 -> Add1/2
  Constant1/1 -> Add2/2
  f_b/1 -> Product1/2, Product4/2, Add4/2
  Add2/1 -> Cos2/1, Cos5/1
  Add4/1 -> Gain3/1
  Product3/1 -> Add3/1
  Product2/1 -> Add/3
  Gain3/1 -> f_0/1
  Cos3/1 -> Product3/1
  Add3/1 -> Gain1/1
  Gain1/1 -> f_d/1
  Product1/1 -> Add/2
  Cos/1 -> Product/1
  Cos1/1 -> Product1/1
  Product4/1 -> Add3/2

== system SistemaCompleto_PMSM/Modelo Global NL perfil trapezoidal aceleracion1/Planta/Subsistema Electromagnetico ==
  v_qs : Inport
  v_ds : Inport  Port=2
  v_0s : Inport  Port=3
  ωm : Inport  Port=4
  R_s(T(t)) : Inport  Port=5
  Add : Sum  Inputs=-++
  Add1 : Sum  Inputs=--+
  Add2 : Sum  Inputs=|-+
  Add3 : Sum  Inputs=|++
  Gain : Gain  Gain=1/L_q
  Gain1 : Gain  Gain=1/L_d
  Gain2 : Gain  Gain=1/L_ls
  Gain3 : Gain  Gain=P_p
  Gain4 : Gain  Gain=L_d
  Gain5 : Gain  Gain=L_q
  Gain6 : Gain  Gain=3/2*P_p
  Gain7 : Gain  Gain=L_d-L_q
  Integrator : Integrator
  Integrator1 : Integrator  InitialCondition=i_ds_inicial
  Integrator2 : Integrator
  Product{,1..6} (7 alike) : Product
  Sum3 : Sum  Inputs=|++
  λ : Constant  Value=lambda_r
  i_qs : Outport
  i_ds : Outport  Port=2
  i_0s : Outport  Port=3
  T_m : Outport  Port=4
  wires:
  v_0s/1 -> Add2/2
  Gain5/1 -> Add/3
  Gain3/1 -> Product4/2, Product3/1  "ωr"
  Integrator/1 -> Product4/1, Product/2, i_qs/1, Product5/1, Product6/1
  v_qs/1 -> Add1/3
  R_s(T(t))/1 -> Product2/2, Product1/1, Product/1
  Gain4/1 -> Sum3/1
  Product1/1 -> Add/1
  Integrator2/1 -> i_0s/1, Product2/1
  Sum3/1 -> Product3/2
  Integrator1/1 -> Gain4/1, Product1/2, i_ds/1, Product6/2
  Product/1 -> Add1/2
  Product4/1 -> Gain5/1
  ωm/1 -> Gain3/1
  Add3/1 -> Gain6/1
  Gain/1 -> Integrator/1
  Gain6/1 -> T_m/1
  Product2/1 -> Add2/1
  λ/1 -> Sum3/2, Product5/2
  Gain1/1 -> Integrator1/1
  Add/1 -> Gain1/1
  Add1/1 -> Gain/1
  Product6/1 -> Gain7/1
  Product3/1 -> Add1/1
  Gain2/1 -> Integrator2/1
  Gain7/1 -> Add3/2
  v_ds/1 -> Add/2
  Add2/1 -> Gain2/1
  Product5/1 -> Add3/1

== system SistemaCompleto_PMSM/Modelo Global NL perfil trapezoidal aceleracion1/Planta/Subsistema Mecanico ==
  Tld(t)[N.m] : Inport
  Tm(t)[N.m] : Inport  Port=2
  1/J_eq[kg.m2] : Gain  Gain=1/J_eq
  Gain : Gain  Gain=1/r
  Gain1 : Gain  Gain=1/r
  Integrator : Integrator  InitialCondition=pos_inicial*r
  Integrator1 : Integrator
  Sin : Trigonometry
  Sum : Sum  Inputs=-+-
  Sum1 : Sum
  "[N.m/rad]" : Gain  Gain=g*k_l
  b_eq[N.m/rad/s] : Gain  Gain=b_eq
  θm(t) : Outport
  ωm(t) : Outport  Port=2
  wires:
  Gain1/1 -> Sin/1
  Sin/1 -> "[N.m/rad]"/1  "θm[rad]"
  Integrator1/1 -> Integrator/1, ωm(t)/1, b_eq[N.m/rad/s]/1  "ωm[rad/s]"
  Tld(t)[N.m]/1 -> Sum1/1
  b_eq[N.m/rad/s]/1 -> Sum/3
  1/J_eq[kg.m2]/1 -> Integrator1/1  "dω/dt [rad/s^2]"
  Gain/1 -> Sum/1
  "[N.m/rad]"/1 -> Sum1/2
  Integrator/1 -> θm(t)/1, Gain1/1  "θm[rad]"
  Sum/1 -> 1/J_eq[kg.m2]/1
  Tm(t)[N.m]/1 -> Sum/2
  Sum1/1 -> Gain/1

== system SistemaCompleto_PMSM/Modelo Global NL perfil trapezoidal aceleracion1/Planta/Subsistema Térmico ==
  i_qs2 : Inport
  i_ds2 : Inport  Port=2
  i_0s2 : Inport  Port=3
  Add : Sum  Inputs=+-
  Add1 : Sum
  Add2 : Sum  Inputs=+++
  Add3 : Sum  Inputs=+-
  Add4 : Sum  Inputs=-+
  Constant : Constant  Value=T_sREF
  Constant1 : Constant
  Constant2 : Constant  Value=T_amb
  Gain : Gain  Gain=R_sREF
  Gain1 : Gain  Gain=a_cu
  Gain2 : Gain  Gain=3/2
  Gain3 : Gain  Gain=2
  Gain4 : Gain  Gain=1/C_ts
  Gain5 : Gain  Gain=1/R_ts_amb
  Integrator : Integrator  InitialCondition=T_amb
  Product : Product
  Square : Math  Operator=square  OutDataTypeStr=double
  Square1 : Math  Operator=square
  Square2 : Math  Operator=square
  R_s : Outport
  T_s : Outport  Port=2
  wires:
  Constant1/1 -> Add1/2
  Constant/1 -> Add/2
  i_qs2/1 -> Square/1
  Gain/1 -> R_s/1, Product/1
  Square/1 -> Add2/1
  Add2/1 -> Gain2/1
  Constant2/1 -> Add4/1
  i_ds2/1 -> Square1/1
  Gain5/1 -> Add3/2
  Integrator/1 -> Add4/2, T_s/1, Add/1  "T_s"
  Add1/1 -> Gain/1
  i_0s2/1 -> Square2/1
  Square1/1 -> Add2/2
  Product/1 -> Add3/1  "Ps_Perd"
  Gain2/1 -> Product/2
  Add/1 -> Gain1/1
  Square2/1 -> Gain3/1
  Gain1/1 -> Add1/1
  Add3/1 -> Gain4/1
  Add4/1 -> Gain5/1
  Gain3/1 -> Add2/3
  Gain4/1 -> Integrator/1

== system SistemaCompleto_PMSM/Modelo Global NL perfil trapezoidal aceleracion1/Planta/TI de Park ==
  f_q : Inport
  f_d : Inport  Port=2
  f_0 : Inport  Port=3
  θ_r : Inport  Port=4
  Add : Sum  Inputs=+++
  Add1 : Sum  Inputs=+-
  Add2 : Sum
  Add3 : Sum  Inputs=+++
  Add4 : Sum  Inputs=+++
  Constant : Constant  Value=2/3*pi
  Constant1 : Constant  Value=2/3*pi
  Cos : Trigonometry  Operator=cos
  Cos1 : Trigonometry
  Cos2 : Trigonometry  Operator=cos
  Cos3 : Trigonometry  Operator=cos
  Cos4 : Trigonometry
  Cos5 : Trigonometry
  Product{,1..5} (6 alike) : Product
  f_a : Outport
  f_b : Outport  Port=2
  f_c : Outport  Port=3
  wires:
  Product4/1 -> Add3/2
  Cos1/1 -> Product1/1
  Cos/1 -> Product/1
  Product1/1 -> Add/2
  Add3/1 -> f_b/1
  Cos3/1 -> Product3/1
  Product3/1 -> Add3/1
  f_d/1 -> Product1/2, Product5/2, Product4/2
  Constant1/1 -> Add2/2
  Constant/1 -> Add1/2
  f_0/1 -> Add3/3, Add4/3, Add/3
  Add1/1 -> Cos3/1, Cos4/1
  Product/1 -> Add/1
  f_q/1 -> Product/2, Product2/2, Product3/2
  Cos4/1 -> Product4/1
  θ_r/1 -> Add2/1, Add1/1, Cos/1, Cos1/1
  Add/1 -> f_a/1
  Add4/1 -> f_c/1
  Cos2/1 -> Product2/1
  Cos5/1 -> Product5/1
  Add2/1 -> Cos5/1, Cos2/1
  Product2/1 -> Add4/1
  Product5/1 -> Add4/2

== system SistemaCompleto_PMSM/Modelo Global NL perfil trapezoidal aceleracion1/Planta/Transformacion de Park ==
  f_a : Inport
  f_b : Inport  Port=2
  f_c : Inport  Port=3
  θ_r : Inport  Port=4
  Add : Sum  Inputs=+++
  Add1 : Sum  Inputs=+-
  Add2 : Sum
  Add3 : Sum  Inputs=+++
  Add4 : Sum  Inputs=+++
  Constant : Constant  Value=2/3*pi
  Constant1 : Constant  Value=2/3*pi
  Cos : Trigonometry  Operator=cos
  Cos1 : Trigonometry  Operator=cos
  Cos2 : Trigonometry  Operator=cos
  Cos3 : Trigonometry
  Cos4 : Trigonometry
  Cos5 : Trigonometry
  Gain1 : Gain  Gain=2/3
  Gain2 : Gain  Gain=2/3
  Gain3 : Gain  Gain=1/3
  Product{,1..5} (6 alike) : Product
  f_q : Outport
  f_d : Outport  Port=2
  f_0 : Outport  Port=3
  wires:
  Cos5/1 -> Product5/1
  Gain2/1 -> f_q/1
  Product5/1 -> Add3/3
  Add/1 -> Gain2/1
  θ_r/1 -> Cos3/1, Cos/1, Add1/1, Add2/1
  Cos4/1 -> Product4/1
  Cos2/1 -> Product2/1
  f_a/1 -> Add4/3, Product3/2, Product/2
  Product/1 -> Add/1
  Add1/1 -> Cos1/1, Cos4/1
  f_c/1 -> Product2/2, Product5/2, Add4/1
  Constant/1 -> Add1/2
  Constant1/1 -> Add2/2
  f_b/1 -> Product1/2, Product4/2, Add4/2
  Add2/1 -> Cos2/1, Cos5/1
  Add4/1 -> Gain3/1
  Product3/1 -> Add3/1
  Product2/1 -> Add/3
  Gain3/1 -> f_0/1
  Cos3/1 -> Product3/1
  Add3/1 -> Gain1/1
  Gain1/1 -> f_d/1
  Product1/1 -> Add/2
  Cos/1 -> Product/1
  Cos1/1 -> Product1/1
  Product4/1 -> Add3/2

== system SistemaCompleto_PMSM/Modelo Global NL perfil trapezoidal aceleracion2/Controlador PID de Posicion/Integrador Tustin ==
  Actual : Inport
  Gain : Gain  Gain=T_s/2
  Sum : Sum  Inputs=|++
  Sum2 : Sum  Inputs=++|
  Unit Delay : UnitDelay  SampleTime=T_s  HasFrameUpgradeWarning=on
  Unit Delay1 : UnitDelay  SampleTime=T_s  HasFrameUpgradeWarning=on
  Int : Outport
  wires:
  Actual/1 -> Unit Delay/1, Sum2/2  "x[n]"
  Sum2/1 -> Gain/1
  Unit Delay/1 -> Sum2/1  "x[n-1]"
  Gain/1 -> Sum/1
  Unit Delay1/1 -> Int/1, Sum/2  "y[n-1]"
  Sum/1 -> Unit Delay1/1  "y[n]"

== system SistemaCompleto_PMSM/Modelo Global NL perfil trapezoidal aceleracion2/Controlador PID de Posicion/Integrador Tustin1 ==
  Actual : Inport
  Gain : Gain  Gain=T_s/2
  Sum : Sum  Inputs=|++
  Sum2 : Sum  Inputs=++|
  Unit Delay : UnitDelay  SampleTime=T_s  HasFrameUpgradeWarning=on
  Unit Delay1 : UnitDelay  SampleTime=T_s  HasFrameUpgradeWarning=on
  Int : Outport
  wires:
  Actual/1 -> Unit Delay/1, Sum2/2  "x[n]"
  Sum2/1 -> Gain/1
  Unit Delay/1 -> Sum2/1  "x[n-1]"
  Gain/1 -> Sum/1
  Unit Delay1/1 -> Int/1, Sum/2  "y[n-1]"
  Sum/1 -> Unit Delay1/1  "y[n]"

== system SistemaCompleto_PMSM/Modelo Global NL perfil trapezoidal aceleracion2/Observador de Estado de velocidad /Integrador Tustin1 ==
  Actual : Inport
  Gain : Gain  Gain=T_s/2
  Sum : Sum  Inputs=|++
  Sum2 : Sum  Inputs=++|
  Unit Delay : UnitDelay  SampleTime=T_s  HasFrameUpgradeWarning=on
  Unit Delay1 : UnitDelay  SampleTime=T_s  HasFrameUpgradeWarning=on
  Int : Outport
  wires:
  Actual/1 -> Unit Delay/1, Sum2/2  "x[n]"
  Sum2/1 -> Gain/1
  Unit Delay/1 -> Sum2/1  "x[n-1]"
  Gain/1 -> Sum/1
  Unit Delay1/1 -> Int/1, Sum/2  "y[n-1]"
  Sum/1 -> Unit Delay1/1  "y[n]"

== system SistemaCompleto_PMSM/Modelo Global NL perfil trapezoidal aceleracion2/Observador de Estado de velocidad /Integrador Tustin2 ==
  Actual : Inport
  Gain : Gain  Gain=T_s/2
  Sum : Sum  Inputs=|++
  Sum2 : Sum  Inputs=++|
  Unit Delay : UnitDelay  SampleTime=T_s  HasFrameUpgradeWarning=on
  Unit Delay1 : UnitDelay  SampleTime=T_s  HasFrameUpgradeWarning=on
  Int : Outport
  wires:
  Actual/1 -> Unit Delay/1, Sum2/2  "x[n]"
  Sum2/1 -> Gain/1
  Unit Delay/1 -> Sum2/1  "x[n-1]"
  Gain/1 -> Sum/1
  Unit Delay1/1 -> Int/1, Sum/2  "y[n-1]"
  Sum/1 -> Unit Delay1/1  "y[n]"

== system SistemaCompleto_PMSM/Modelo Global NL perfil trapezoidal aceleracion2/Observador de Estado de velocidad /Integrador Tustin3 ==
  Actual : Inport
  Gain : Gain  Gain=T_s/2
  Sum : Sum  Inputs=|++
  Sum2 : Sum  Inputs=++|
  Unit Delay : UnitDelay  SampleTime=T_s  HasFrameUpgradeWarning=on
  Unit Delay1 : UnitDelay  SampleTime=T_s  HasFrameUpgradeWarning=on
  Int : Outport
  wires:
  Actual/1 -> Unit Delay/1, Sum2/2  "x[n]"
  Sum2/1 -> Gain/1
  Unit Delay/1 -> Sum2/1  "x[n-1]"
  Gain/1 -> Sum/1
  Unit Delay1/1 -> Int/1, Sum/2  "y[n-1]"
  Sum/1 -> Unit Delay1/1  "y[n]"

== system SistemaCompleto_PMSM/Modelo Global NL perfil trapezoidal aceleracion2/Planta/Subsistema Electromagnetico ==
  v_qs : Inport
  v_ds : Inport  Port=2
  v_0s : Inport  Port=3
  ωm : Inport  Port=4
  R_s(T(t)) : Inport  Port=5
  Add : Sum  Inputs=-++
  Add1 : Sum  Inputs=--+
  Add2 : Sum  Inputs=|-+
  Add3 : Sum  Inputs=|++
  Gain : Gain  Gain=1/L_q
  Gain1 : Gain  Gain=1/L_d
  Gain2 : Gain  Gain=1/L_ls
  Gain3 : Gain  Gain=P_p
  Gain4 : Gain  Gain=L_d
  Gain5 : Gain  Gain=L_q
  Gain6 : Gain  Gain=3/2*P_p
  Gain7 : Gain  Gain=L_d-L_q
  Integrator : Integrator
  Integrator1 : Integrator  InitialCondition=i_ds_inicial
  Integrator2 : Integrator
  Product{,1..6} (7 alike) : Product
  Sum3 : Sum  Inputs=|++
  λ : Constant  Value=lambda_r
  i_qs : Outport
  i_ds : Outport  Port=2
  i_0s : Outport  Port=3
  T_m : Outport  Port=4
  wires:
  Product5/1 -> Add3/1
  Add2/1 -> Gain2/1
  v_ds/1 -> Add/2
  Gain7/1 -> Add3/2
  Gain2/1 -> Integrator2/1
  Product3/1 -> Add1/1
  Product6/1 -> Gain7/1
  Add1/1 -> Gain/1
  Add/1 -> Gain1/1
  Gain1/1 -> Integrator1/1
  λ/1 -> Product5/2, Sum3/2
  Product2/1 -> Add2/1
  Gain6/1 -> T_m/1
  Gain/1 -> Integrator/1
  Add3/1 -> Gain6/1
  ωm/1 -> Gain3/1
  Product4/1 -> Gain5/1
  Product/1 -> Add1/2
  Integrator1/1 -> Product6/2, i_ds/1, Product1/2, Gain4/1
  Sum3/1 -> Product3/2
  Integrator2/1 -> Product2/1, i_0s/1
  Product1/1 -> Add/1
  Gain4/1 -> Sum3/1
  R_s(T(t))/1 -> Product/1, Product1/1, Product2/2
  v_qs/1 -> Add1/3
  Integrator/1 -> Product6/1, Product5/1, i_qs/1, Product/2, Product4/1
  Gain3/1 -> Product3/1, Product4/2  "ωr"
  Gain5/1 -> Add/3
  v_0s/1 -> Add2/2

== system SistemaCompleto_PMSM/Modelo Global NL perfil trapezoidal aceleracion2/Planta/Subsistema Mecanico ==
  Tld(t)[N.m] : Inport
  Tm(t)[N.m] : Inport  Port=2
  g [m/s2] : Inport  Port=3
  1/J_eq[kg.m2] : Gain  Gain=1/J_eq
  Gain : Gain  Gain=1/r
  Gain1 : Gain  Gain=1/r
  Integrator : Integrator  InitialCondition=pos_inicial*r
  Integrator1 : Integrator
  Product : Product
  Sin : Trigonometry
  Sum : Sum  Inputs=-+-
  Sum1 : Sum
  "[N.m/rad]" : Gain  Gain=k_l
  b_eq[N.m/rad/s] : Gain  Gain=b_eq
  θm(t) : Outport
  ωm(t) : Outport  Port=2
  wires:
  g [m/s2]/1 -> Product/1
  "[N.m/rad]"/1 -> Product/2
  Integrator1/1 -> Integrator/1, ωm(t)/1, b_eq[N.m/rad/s]/1  "ωm[rad/s]"
  Gain1/1 -> Sin/1
  Tld(t)[N.m]/1 -> Sum1/1
  b_eq[N.m/rad/s]/1 -> Sum/3
  Gain/1 -> Sum/1
  Integrator/1 -> Gain1/1, θm(t)/1  "θm[rad]"
  Sum/1 -> 1/J_eq[kg.m2]/1
  1/J_eq[kg.m2]/1 -> Integrator1/1  "dω/dt [rad/s^2]"
  Sin/1 -> "[N.m/rad]"/1  "θm[rad]"
  Sum1/1 -> Gain/1
  Product/1 -> Sum1/2
  Tm(t)[N.m]/1 -> Sum/2

== system SistemaCompleto_PMSM/Modelo Global NL perfil trapezoidal aceleracion2/Planta/Subsistema Térmico ==
  i_qs2 : Inport
  i_ds2 : Inport  Port=2
  i_0s2 : Inport  Port=3
  Add : Sum  Inputs=+-
  Add1 : Sum
  Add2 : Sum  Inputs=+++
  Add3 : Sum  Inputs=+-
  Add4 : Sum  Inputs=-+
  Constant : Constant  Value=T_sREF
  Constant1 : Constant
  Constant2 : Constant  Value=T_amb
  Gain : Gain  Gain=R_sREF
  Gain1 : Gain  Gain=a_cu
  Gain2 : Gain  Gain=3/2
  Gain3 : Gain  Gain=2
  Gain4 : Gain  Gain=1/C_ts
  Gain5 : Gain  Gain=1/R_ts_amb
  Integrator : Integrator  InitialCondition=T_amb
  Product : Product
  Square : Math  Operator=square  OutDataTypeStr=double
  Square1 : Math  Operator=square
  Square2 : Math  Operator=square
  R_s : Outport
  T_s : Outport  Port=2
  wires:
  Gain4/1 -> Integrator/1
  Gain3/1 -> Add2/3
  Add4/1 -> Gain5/1
  Add3/1 -> Gain4/1
  Gain1/1 -> Add1/1
  Square2/1 -> Gain3/1
  Add/1 -> Gain1/1
  Gain2/1 -> Product/2
  Product/1 -> Add3/1  "Ps_Perd"
  Square1/1 -> Add2/2
  i_0s2/1 -> Square2/1
  Add1/1 -> Gain/1
  Integrator/1 -> Add/1, T_s/1, Add4/2  "T_s"
  Gain5/1 -> Add3/2
  i_ds2/1 -> Square1/1
  Constant2/1 -> Add4/1
  Add2/1 -> Gain2/1
  Square/1 -> Add2/1
  Gain/1 -> Product/1, R_s/1
  i_qs2/1 -> Square/1
  Constant/1 -> Add/2
  Constant1/1 -> Add1/2

== system SistemaCompleto_PMSM/Modelo Global NL perfil trapezoidal aceleracion2/Planta/TI de Park ==
  f_q : Inport
  f_d : Inport  Port=2
  f_0 : Inport  Port=3
  θ_r : Inport  Port=4
  Add : Sum  Inputs=+++
  Add1 : Sum  Inputs=+-
  Add2 : Sum
  Add3 : Sum  Inputs=+++
  Add4 : Sum  Inputs=+++
  Constant : Constant  Value=2/3*pi
  Constant1 : Constant  Value=2/3*pi
  Cos : Trigonometry  Operator=cos
  Cos1 : Trigonometry
  Cos2 : Trigonometry  Operator=cos
  Cos3 : Trigonometry  Operator=cos
  Cos4 : Trigonometry
  Cos5 : Trigonometry
  Product{,1..5} (6 alike) : Product
  f_a : Outport
  f_b : Outport  Port=2
  f_c : Outport  Port=3
  wires:
  Product5/1 -> Add4/2
  Product2/1 -> Add4/1
  Add2/1 -> Cos2/1, Cos5/1
  Cos5/1 -> Product5/1
  Cos2/1 -> Product2/1
  Add4/1 -> f_c/1
  Add/1 -> f_a/1
  θ_r/1 -> Cos1/1, Cos/1, Add1/1, Add2/1
  Cos4/1 -> Product4/1
  f_q/1 -> Product3/2, Product2/2, Product/2
  Product/1 -> Add/1
  Add1/1 -> Cos4/1, Cos3/1
  f_0/1 -> Add/3, Add4/3, Add3/3
  Constant/1 -> Add1/2
  Constant1/1 -> Add2/2
  f_d/1 -> Product4/2, Product5/2, Product1/2
  Product3/1 -> Add3/1
  Cos3/1 -> Product3/1
  Add3/1 -> f_b/1
  Product1/1 -> Add/2
  Cos/1 -> Product/1
  Cos1/1 -> Product1/1
  Product4/1 -> Add3/2
